simulink model "mymodel2"  (R2020a)
settings: Solver=VariableStepAuto  StartTime=0.0  StopTime=10.0  RelTol=1e-3
libraries: fuzblock x1
settings Model: Creator=Aman's Notebook  LastModifiedBy=Aman's Notebook

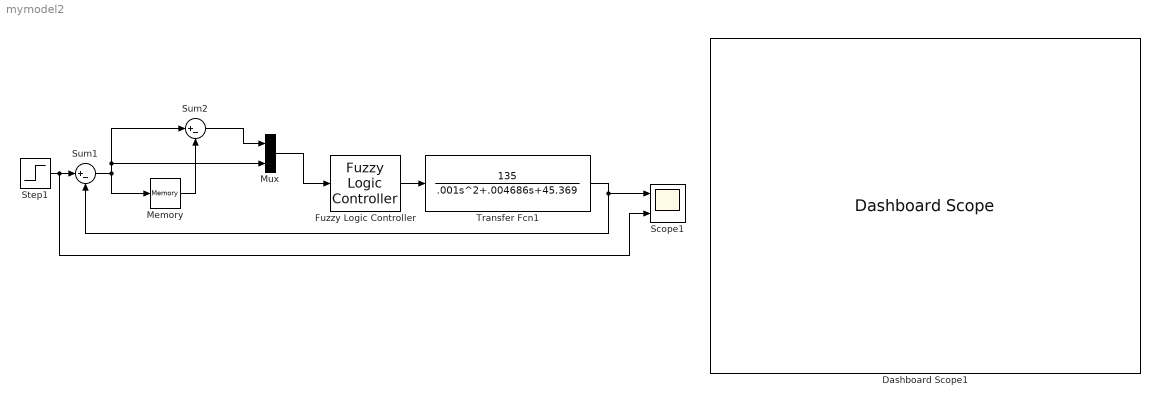
== system mymodel2 ==
  Dashboard Scope1 : DashboardScope
  Fuzzy Logic Controller : fuzblock/Fuzzy Logic  Controller  FIS=fpid_controller  OutputSampleNumber=101  DataType=double  FuzzifiedInputs=off  RuleFiringStrengths=off  RuleOutputs=off  AggregatedOutputs=off  SimulateUsing=Interpreted execution  OutOfRangeInputValueMessage=warning  NoRuleFiredMessage=warning  EmptyOutputFuzzySetMessage=warning
  Memory : Memory
  Mux : Mux  Inputs=2
  Scope1 : Scope  NumInputPorts=2
  Step1 : Step  SampleTime=0
  Sum1 : Sum  Inputs=|+-
  Sum2 : Sum  Inputs=|+-
  Transfer Fcn1 : TransferFcn  Numerator=[135]  Denominator=[.001 .004686 45.369]
  wires:
  Step1/1 -> Sum1/1, Scope1/2
  Fuzzy Logic Controller/1 -> Transfer Fcn1/1
  Transfer Fcn1/1 -> Scope1/1, Sum1/2
  Sum1/1 -> Sum2/1, Mux/2, Memory/1
  Memory/1 -> Sum2/2
  Sum2/1 -> Mux/1
  Mux/1 -> Fuzzy Logic Controller/1
